simulink model "push_set_reset"  (R2021a)
settings: Solver=VariableStepAuto  StartTime=0.0  StopTime=inf  RelTol=1e-3
libraries: simulink x1
settings Model: Creator=surya  LastModifiedBy=surya

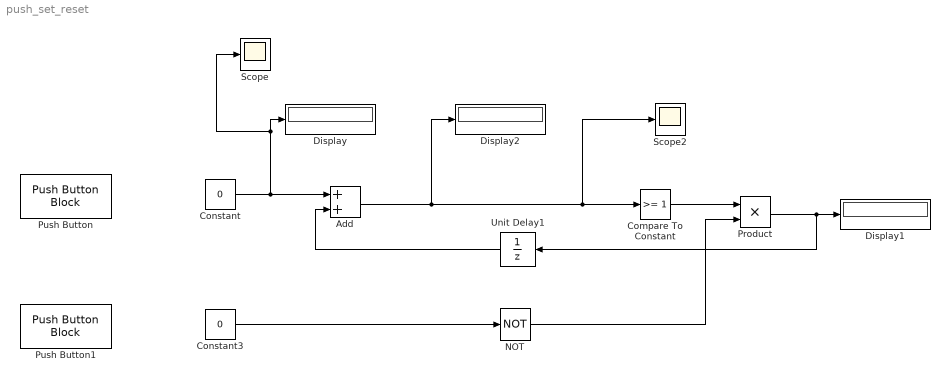
== system push_set_reset ==
  Add : Sum
  Compare To Constant : simulink/Logic and Bit Operations/Compare To Constant  relop=>=  const=1  OutDataTypeStr=boolean
  Constant : Constant  Value=0
  Constant3 : Constant  Value=0  OutDataTypeStr=boolean
  Display : Display
  Display1 : Display
  Display2 : Display
  NOT : Logic  Operator=NOT  IconShape=distinctive  AllPortsSameDT=off  OutDataTypeStr=boolean
  Product : Product  OutDataTypeStr=double
  Push Button : PushButtonBlock  ButtonText=set
  Push Button1 : PushButtonBlock  ButtonText=reset
  Scope : Scope
  Scope2 : Scope
  Unit Delay1 : UnitDelay  HasFrameUpgradeWarning=on
  wires:
  Constant/1 -> Add/1, Display/1, Scope/1
  Unit Delay1/1 -> Add/2
  Add/1 -> Scope2/1, Compare To Constant/1, Display2/1
  Constant3/1 -> NOT/1
  NOT/1 -> Product/2
  Product/1 -> Unit Delay1/1, Display1/1
  Compare To Constant/1 -> Product/1
